simulink model "CDC2019Preisach"  (R2020a)
settings: Solver=FixedStepAuto  StartTime=0.0  StopTime=simTotalTime  FixedStep=0.05  MaxStep=0.1  MinStep=0.01  RelTol=1e-3
undefined symbols (not defined in the file): CA, CB, CC, CD, Cx0, GA, GB, GC, GD, gridSize, Gx0, initialRelays, inputAmp, inputFactor, inputGrid, inputMax, inputMin, offset, outputAmp, outputFactor, outputMax, outputMin, relayArea, relayLength, relayOffVal, relayOnVal, weightFunc
libraries: simulink x1
settings Model: Creator=Marco  LastModifiedBy=mvasq
settings DataIOCC: ReturnWorkspaceOutputs=off
settings DebuggingCC: ArithmeticOperatorsInVariantConditions=warning
settings SFSimCC: SimUseLocalCustomCode=off  CustomCodeUndefinedFunction=UseInterfaceOnly
settings RTWCC: RTWUseLocalCustomCode=off

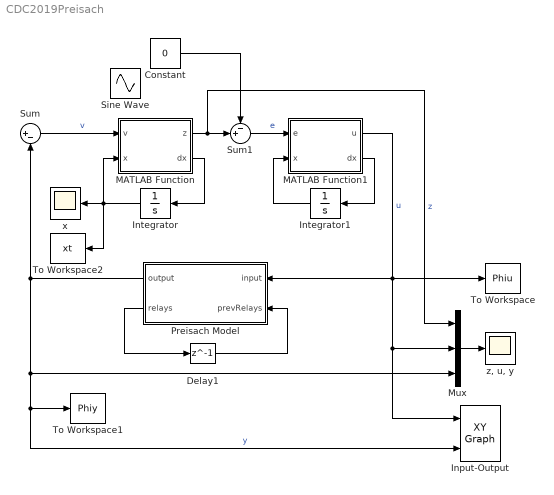
== system CDC2019Preisach ==
  Constant : Constant  Value=0
  Delay1 : Delay  DelayLength=1  InitialCondition=initialRelays
  Input-Output : simulink/Sinks/XY Graph  xmin=inputMin - inputAmp*inputFactor  xmax=inputMax + inputAmp*inputFactor  ymin=outputMin - outputAmp*outputFactor  ymax=outputMax + outputAmp*outputFactor  st=-1
  Integrator : Integrator  InitialCondition=Gx0
  Integrator1 : Integrator  InitialCondition=Cx0
  MATLAB Function : MATLAB Function  TreatAsAtomicUnit=on
  MATLAB Function1 : MATLAB Function  TreatAsAtomicUnit=on
  Mux : Mux  Inputs=3
  Preisach Model : MATLAB Function  TreatAsAtomicUnit=on
  Sine Wave : Sin  Amplitude=0.8  Frequency=2*pi*(1/20)  SampleTime=0
  Sum : Sum  Inputs=|+-
  Sum1 : Sum  Inputs=-+|
  To Workspace : ToWorkspace  VariableName=Phiu  SaveFormat=Timeseries  SampleTime=-1
  To Workspace1 : ToWorkspace  VariableName=Phiy  SaveFormat=Timeseries  SampleTime=-1
  To Workspace2 : ToWorkspace  VariableName=xt  SaveFormat=Timeseries  SampleTime=-1
  x : Scope
  "z, u, y" : Scope
  wires:
  Preisach Model/2(relays) -> Delay1/1
  Delay1/1 -> Preisach Model/2(prevRelays)
  Sum/1 -> MATLAB Function/1(v)  "v"
  Preisach Model/1(output) -> To Workspace1/1, Input-Output/2, Mux/3, Sum/2  "y"
  Mux/1 -> "z, u, y"/1
  MATLAB Function/2(dx) -> Integrator/1
  Integrator/1 -> To Workspace2/1, MATLAB Function/2(x), x/1
  Integrator1/1 -> MATLAB Function1/2(x)
  MATLAB Function1/2(dx) -> Integrator1/1
  MATLAB Function/1(z) -> Sum1/2, Mux/1  "z"
  Sum1/1 -> MATLAB Function1/1(e)  "e"
  MATLAB Function1/1(u) -> To Workspace/1, Input-Output/1, Mux/2, Preisach Model/1(input)  "u"
  Constant/1 -> Sum1/1

== matlab function CDC2019Preisach/MATLAB Function ==
  data: v input; z output; x input; GA parameter; GB parameter; GC parameter; dx output; GD parameter
function [z,dx] = fcn(v, x, GA, GB, GC, GD)

dx = GA*x + GB*v;
z = GC*x + GD*v;

== matlab function CDC2019Preisach/Preisach Model ==
  data: input input; prevRelays input; output output; weightFunc parameter; relays output; offset parameter; relayOffVal parameter; relayOnVal parameter; gridSize parameter; inputGrid parameter; relayLength parameter; relayArea parameter
function [output, relays] = fcn(input, prevRelays, ...
    weightFunc, offset, relayOffVal, relayOnVal, gridSize, inputGrid, relayLength, relayArea)

%     output = offset;
%     relays = prevRelays;
%     for i=1:gridSize
%         ii = gridSize-i+1; %index inversion for rows
%         for j=1:i
%             if( input >= inputGrid(i) && relays(ii,j) ~= relayOnVal )
%                 relays(ii,j) = relayOnVal;
%             elseif( input <= inputGrid(j) && relays(ii,j) ~= relayOffVal )
%                 relays(ii,j) = relayOffVal;
%             end
%             output = output + relays(ii,j)*weightFunc(ii,j)*relayArea;
%         end
%     end


%     relays = prevRelays;
%     for row=1:gridSize+1
%         if( row == gridSize+1 || input <= inputGrid(row) )
%             row = row-1;
%             irow = gridSize-row+1;
%             relays(irow:end, 1:row) = relayOnVal*fliplr(triu(ones(row, row)));
%             break;
%         end
%     end
%     for col=gridSize:-1:0
%         if( col == 0 || input >= inputGrid(col) )
%             col = col+1;
%             irow = gridSize-col+1;
%             relays(1:irow, col:end) = relayOffVal*fliplr(triu(ones(irow, irow)));
%             break;
%         end
%     end
%     output = sum(sum(relays(:,:).*weightFunc(:,:)))*relayArea + offset;


    relays = prevRelays;
    if( inputGrid(end) <= input )
        relays(:,:) = relayOnVal*fliplr(triu(ones(gridSize, gridSize)));
    elseif( input < inputGrid(1) )
        relays(:,:) = relayOffVal*fliplr(triu(ones(gridSize, gridSize)));
    else
        idx0 = 1;
        while( idx0 <= gridSize-1 )
            if( inputGrid(idx0) <= input && input < inputGrid(idx0+1) )
                col = idx0;
                row = gridSize-idx0+1;

                relays(row:end, 1:col) = relayOnVal*fliplr(triu(ones(col, col)));
                relays(1:row-1, col+1:end) = relayOffVal*fliplr(triu(ones(row-1, row-1)));
                break;
            end
            idx0 = idx0 + 1;
        end
    end
    output = sum(sum(relays(:,:).*weightFunc(:,:)))*relayArea + offset;

== matlab function CDC2019Preisach/MATLAB Function1 ==
  data: e input; u output; x input; CA parameter; CB parameter; CC parameter; dx output; CD parameter
function [u, dx] = fcn(e, x, CA, CB, CC, CD)

dx = CA*x + CB*e;
u = CC*x + CD*e;
